simulink model "ADRC_P3DX_Madyan"  (R2024b)
settings: Solver=FixedStepAuto  StartTime=0.0  StopTime=30  FixedStep=0.01  RelTol=1e-2
libraries: simulink x1
settings Model: Creator=Dell  LastModifiedBy=MMadi
settings DebuggingCC: AlgebraicLoopMsg=none  SigSpecEnsureSampleTimeMsg=none
settings RTWCC: GPUComputeCapability=3.5

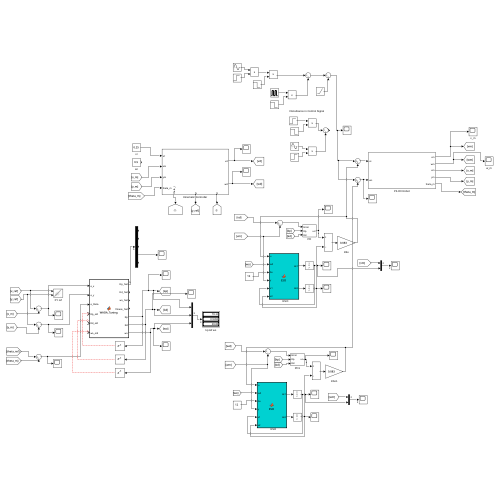
[thumbnail: Simulink's stored preview of the top-level diagram]
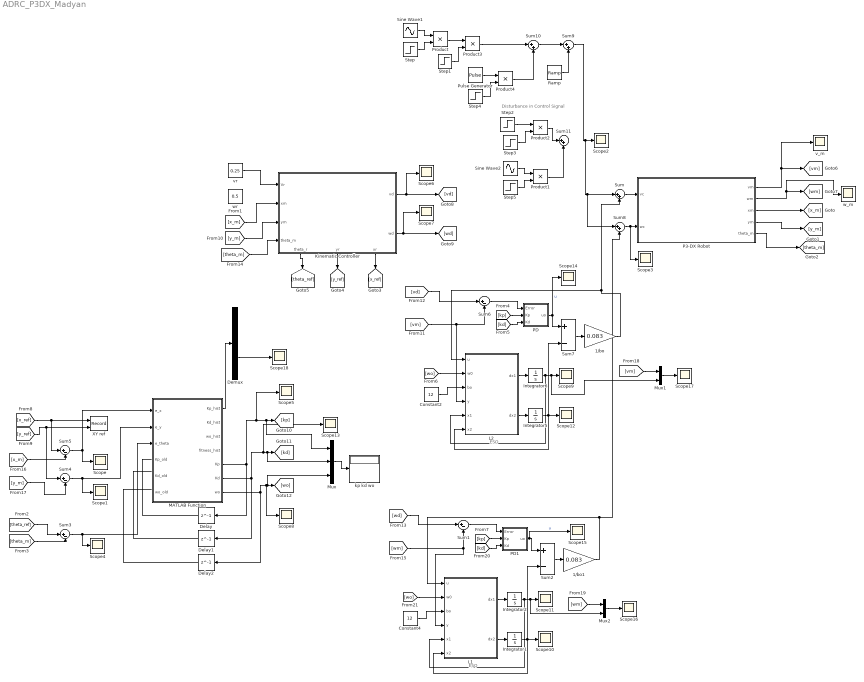
== system ADRC_P3DX_Madyan ==
  note: Disturbance in Control Signal
  note: ESO
  note: ESO
  1/bo : Gain  Gain=0.083
  1/bo1 : Gain  Gain=0.083
  Constant2 : Constant  Value=12
  Constant4 : Constant  Value=12
  Delay : Delay  DelayLength=1  InitialCondition=0
  Delay1 : Delay  DelayLength=1  InitialCondition=0
  Delay2 : Delay  DelayLength=1  InitialCondition=0
  Demux : Demux  Outputs=5
  Integrator{1..2,5..6} (4 alike) : Integrator
  Kinematic Controller : Subsystem
      settings: PortSchema="{\"entries\":[{\"content\":{\"sides\":[{\"content\":{\"connectorIds\":[\"In1\",\"In2\",\"In3\",\"In4\"]},\"type\":\"ConnectorPlacement.EquallySpacedRectSide\",\"uuid\":\"1dde3c4d-b362-4c98-bff5-173134d67a18\"},{\"content\":{\"connectorIds\":[\"Out1\",\"Out2\"],\"side\":\"RIGHT\"},\"type\":\"ConnectorPlacement.EquallySpacedRectSide\",\"uuid\":\"28a7b07a-1542-4ec6-930a-70e18e33702f\"},{\"content\":{\"side\":\"TOP\"},\"type\":\"ConnectorPlacement.EquallySpacedRectSide\",\"uuid\":\"fddfb50e-6b1f-4e7e-bd72-f809cd3d8285\"},{\"content\":{\"connectorIds\":[\"Out3\",\"Out4\",\"Out5\"],\"side\":\"BOTTOM\"},\"type\":\"ConnectorPlacement.EquallySpacedRectSide\",\"uuid\":\"0cbc9f95-9386-4a92-999a-6cc6855b0431\"}]},\"type\":\"ConnectorPlacement.EquallySpacedConnector\",\"uuid\":\"21383b85-61ab-4832-be46-2fedf08e757e\"}],\"packageUris\":[\"http://schema.mathworks.com/mf0/Connector/R2020b\"],\"version\":\"1.0\"}"
  L1 : MATLAB Function  TreatAsAtomicUnit=on
  L2 : MATLAB Function  TreatAsAtomicUnit=on
  MATLAB Function : MATLAB Function  TreatAsAtomicUnit=on
  Mux : Mux  Inputs=3
  Mux1 : Mux  Inputs=2
  Mux2 : Mux  Inputs=2
  P3-DX Robot : Subsystem
  PD : Subsystem
  PD1 : Subsystem
  Product{,1..4} (5 alike) : Product
  Pulse Generator : DiscretePulseGenerator  PulseType=Time based  Amplitude=4  Period=1  PulseWidth=35  PhaseDelay=9.7
  Ramp : simulink/Sources/Ramp  slope=1  start=25  InitialOutput=0
  Scope{,1..18} (19 alike) : Scope
  Sine Wave1 : Sin  Amplitude=4  Frequency=2  SampleTime=0
  Sine Wave2 : Sin  Amplitude=3  Frequency=2  SampleTime=0
  Step : Step  Time=3.2  SampleTime=0
  Step1 : Step  Time=15  Before=1  After=0  SampleTime=0
  Step2 : Step  Time=8  After=1.8  SampleTime=0
  Step3 : Step  Time=10  Before=1.8  After=0  SampleTime=0
  Step4 : Step  Time=23  Before=1  After=0  SampleTime=0
  Step5 : Step  Time=20  SampleTime=0
  Sum{,8..11} (5 alike) : Sum  Inputs=|++
  Sum{1,3..6} (5 alike) : Sum  Inputs=|+-
  Sum2 : Sum  Inputs=+-
  Sum7 : Sum  Inputs=+-
  XY ref : Record  FileSettingsInternal="{\"entries\":[{\"content\":{\"excelSettings\":{\"content\":{},\"type\":\"Streamout.ExcelSettings\"}},\"type\":\"Streamout.FileSettingStorage\",\"uuid\":\"\"}],\"packageUris\":[\"http:\\/\\/schema.mathworks.com\\/mf0\\/streamout_blocks\\/R2020a\"],\"version\":\"1.0\"}"  Layout=[1 1]  SignalsInternal="{\"entries\":[{\"content\":{\"signals\":[{\"content\":{\"blockPath\":[],\"dimensions\":[1],\"domain\":\"\",\"lineColor\":\"#edb120\",\"lineWidth\":2,\"port\":1,\"signalID\":1,\"signalName\":\"From8\"},\"type\":\"RecordBlkView.Signal\",\"uuid\":\"\"},{\"content\":{\"blockPath\":[],\"dimensions\":[1],\"domain\":\"\",\"lineColor\":\"#7e2f8e\",\"lineWidth\":2,\"port\":2,\"signalID\":2,\"signalName\":\"From9\"},\"type\":\"RecordBlkView.Signal\",\"uuid\":\"\"}]},\"type\":\"RecordBlkView.InputSignals\",\"uuid\":\"\"}],\"packageUris\":[\"http:\\/\\/schema.mathworks.com\\/mf0\\/streamout_blocks\\/R2020a\"],\"version\":\"1.0\"}"  VisualizationBindings="{\"xyplotplugin\":{\"info\":[{\"series\":[],\"subplotID\":1}]}}"  CompatibilityTag=XY
  kp kd wo : Display
  v_m : Scope
  vr : Constant  Value=0.25
  w_m : Scope
  wr : Constant  Value=0.5
  wires:
  [y_ref] -> Sum4/1, XY ref/2
  [x_ref] -> Sum5/1, XY ref/1
  [y_m] -> Kinematic Controller/3(ym)
  vr/1 -> Kinematic Controller/1(Vr)
  [x_m] -> Kinematic Controller/2(xm)
  [theta_m] -> Kinematic Controller/4(theta_m)
  P3-DX Robot/3(xm) -> [x_m]
  P3-DX Robot/4(ym) -> [y_m]
  P3-DX Robot/5(theta_m) -> [theta_m]
  Kinematic Controller/5(xr) -> [x_ref]
  Kinematic Controller/4(yr) -> [y_ref]
  Kinematic Controller/3(theta_r) -> [theta_ref]
  Kinematic Controller/2(wd) -> [wd], Scope7/1
  Kinematic Controller/1(vd) -> [vd], Scope6/1
  1/bo/1 -> Sum/2, L2/1(u)
  [vd] -> Sum6/1
  Integrator6/1 -> L2/5(x1), Mux1/2, Scope9/1
  Sum7/1 -> 1/bo/1
  PD/1(uo) -> Sum7/1, Scope14/1  "u"
  [vm] -> Sum6/2, L2/4(y)
  Sum6/1 -> PD/1(Error)
  Integrator5/1 -> Sum7/2, Scope12/1, L2/6(x2)
  L2/2(dx2) -> Integrator5/1
  L2/1(dx1) -> Integrator6/1
  L1/2(dx2) -> Integrator1/1
  Integrator1/1 -> Sum2/2, Scope10/1, L1/6(x2)
  [wm] -> L1/4(y), Sum1/2
  Sum1/1 -> PD1/1(Error)
  Sum2/1 -> 1/bo1/1
  Integrator2/1 -> L1/5(x1), Mux2/2, Scope11/1
  L1/1(dx1) -> Integrator2/1
  [wd] -> Sum1/1
  Constant4/1 -> L1/3(bo)
  PD1/1(uo) -> Scope15/1, Sum2/1  "u"
  1/bo1/1 -> Sum8/2, L1/1(u)
  Sum/1 -> P3-DX Robot/1(vc)
  Sum8/1 -> Scope3/1, P3-DX Robot/2(wc)
  [vm] -> Mux1/1
  Mux1/1 -> Scope17/1
  [wm] -> Mux2/1
  Mux2/1 -> Scope16/1
  Constant2/1 -> L2/3(bo)
  Sine Wave2/1 -> Product1/1
  Step5/1 -> Product1/2
  Step3/1 -> Product2/2
  Step2/1 -> Product2/1
  P3-DX Robot/1(vm) -> v_m/1, [vm]
  P3-DX Robot/2(wm) -> w_m/1, [wm]
  MATLAB Function/6(Kd) -> Scope13/1, Mux/2, [kd], Delay1/1
  MATLAB Function/7(wo) -> Scope8/1, Mux/3, [wo], Delay2/1
  MATLAB Function/5(Kp) -> Scope5/1, Mux/1, [kp], Delay/1
  [theta_ref] -> Sum3/1
  [theta_m] -> Sum3/2
  [y_m] -> Sum4/2
  [x_m] -> Sum5/2
  Sum5/1 -> Scope/1, MATLAB Function/1(e_x)
  Sum4/1 -> Scope1/1, MATLAB Function/2(e_y)
  Sum3/1 -> Scope4/1, MATLAB Function/3(e_theta)
  [kp] -> PD/2(Kp)
  [kd] -> PD/3(Kd)
  [wo] -> L2/2(w0)
  Delay/1 -> ?
  Delay1/1 -> ?
  Delay2/1 -> ?
  Mux/1 -> kp kd wo/1
  [kp] -> PD1/2(Kp)
  [kd] -> PD1/3(Kd)
  [wo] -> L1/2(w0)
  Product1/1 -> Sum11/2
  Product2/1 -> Sum11/1
  Product3/1 -> Sum10/1
  Pulse Generator/1 -> Product4/1
  Step/1 -> Product/2
  Ramp/1 -> Sum9/2
  Sum10/1 -> Sum9/1
  Product/1 -> Product3/1
  Step1/1 -> Product3/2
  Sine Wave1/1 -> Product/1
  Product4/1 -> Sum10/2
  Step4/1 -> Product4/2
  Sum9/1 -> Sum8/1, Sum/1, Scope2/1
  Demux/4 -> Scope18/1
  MATLAB Function/1(Kp_hist) -> Demux/1

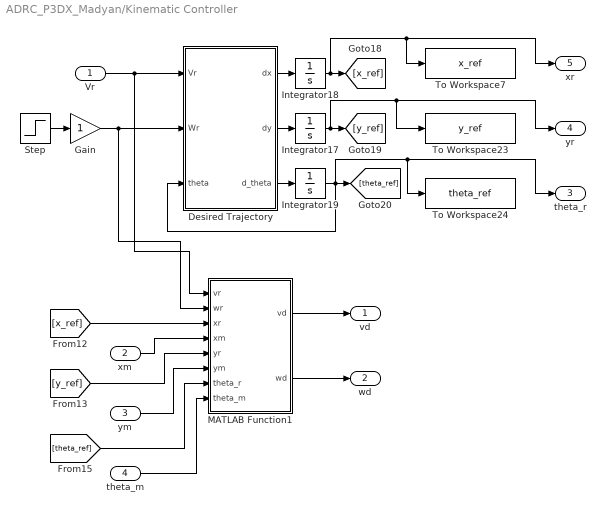
== system ADRC_P3DX_Madyan/Kinematic Controller ==
  Vr : Inport
  xm : Inport  Port=2
  ym : Inport  Port=3
  theta_m : Inport  Port=4
  " Desired Trajectory" : MATLAB Function  TreatAsAtomicUnit=on
  Gain : Gain
  Integrator17 : Integrator  InitialCondition=-0.5
  Integrator18 : Integrator
  Integrator19 : Integrator
  MATLAB Function1 : MATLAB Function  TreatAsAtomicUnit=on
  Step : Step  Time=16  Before=0.5  After=0.4  SampleTime=0
  To Workspace23 : ToWorkspace  VariableName=y_ref  SaveFormat=Timeseries  SampleTime=-1
  To Workspace24 : ToWorkspace  VariableName=theta_ref  SaveFormat=Timeseries  SampleTime=-1
  To Workspace7 : ToWorkspace  VariableName=x_ref  SaveFormat=Timeseries  SampleTime=-1
  vd : Outport
  wd : Outport  Port=2
  theta_r : Outport  Port=3
  yr : Outport  Port=4
  xr : Outport  Port=5
  wires:
  " Desired Trajectory"/3(d_theta) -> Integrator19/1
  Integrator19/1 -> theta_r/1, To Workspace24/1, " Desired Trajectory"/3(theta), [theta_ref]
  Integrator18/1 -> xr/1, To Workspace7/1, [x_ref]
  Vr/1 -> MATLAB Function1/1(vr), " Desired Trajectory"/1(Vr)
  " Desired Trajectory"/1(dx) -> Integrator18/1
  Gain/1 -> MATLAB Function1/2(wr), " Desired Trajectory"/2(Wr)
  MATLAB Function1/1(vd) -> vd/1
  MATLAB Function1/2(wd) -> wd/1
  " Desired Trajectory"/2(dy) -> Integrator17/1
  Integrator17/1 -> yr/1, To Workspace23/1, [y_ref]
  [x_ref] -> MATLAB Function1/3(xr)
  xm/1 -> MATLAB Function1/4(xm)
  [y_ref] -> MATLAB Function1/5(yr)
  ym/1 -> MATLAB Function1/6(ym)
  [theta_ref] -> MATLAB Function1/7(theta_r)
  theta_m/1 -> MATLAB Function1/8(theta_m)
  Step/1 -> Gain/1

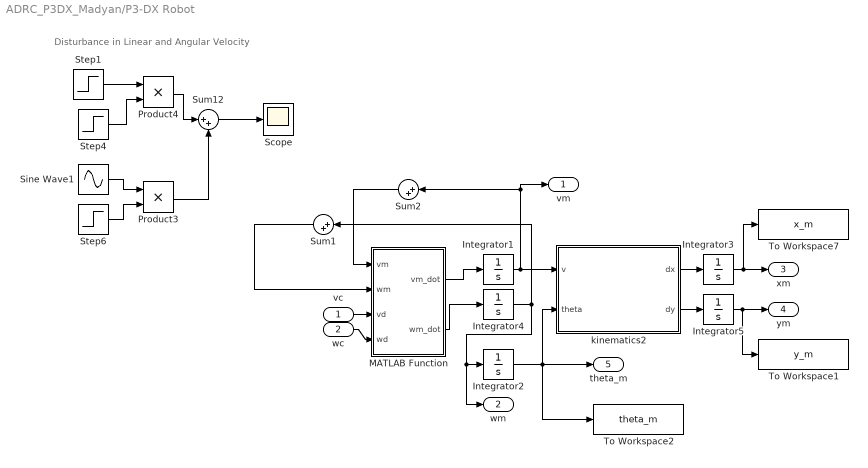
== system ADRC_P3DX_Madyan/P3-DX Robot ==
  note: Disturbance in Linear and Angular Velocity
  vc : Inport
  wc : Inport  Port=2
  Integrator{1..5} (5 alike) : Integrator
  MATLAB Function : MATLAB Function  TreatAsAtomicUnit=on
  Product3 : Product
  Product4 : Product
  Scope : Scope
  Sine Wave1 : Sin  Amplitude=4  Frequency=2  SampleTime=0
  Step1 : Step  Time=8  After=2.2  SampleTime=0
  Step4 : Step  Time=10  Before=2.2  After=0  SampleTime=0
  Step6 : Step  Time=20  SampleTime=0
  Sum1 : Sum  Inputs=|++
  Sum12 : Sum  Inputs=|++
  Sum2 : Sum  Inputs=|++
  To Workspace1 : ToWorkspace  VariableName=y_m  SaveFormat=Timeseries  SampleTime=-1
  To Workspace2 : ToWorkspace  VariableName=theta_m  SaveFormat=Timeseries  SampleTime=-1
  To Workspace7 : ToWorkspace  VariableName=x_m  SaveFormat=Timeseries  SampleTime=-1
  kinematics2 : MATLAB Function  TreatAsAtomicUnit=on
  vm : Outport
  wm : Outport  Port=2
  xm : Outport  Port=3
  ym : Outport  Port=4
  theta_m : Outport  Port=5
  wires:
  Integrator2/1 -> To Workspace2/1, theta_m/1, kinematics2/2(theta)
  MATLAB Function/1(vm_dot) -> Integrator1/1
  MATLAB Function/2(wm_dot) -> Integrator4/1
  Integrator1/1 -> kinematics2/1(v), Sum2/1, vm/1
  Integrator3/1 -> To Workspace7/1, xm/1
  Integrator4/1 -> Integrator2/1, wm/1, Sum1/1
  kinematics2/2(dy) -> Integrator5/1
  vc/1 -> MATLAB Function/3(vd)
  kinematics2/1(dx) -> Integrator3/1
  wc/1 -> MATLAB Function/4(wd)
  Integrator5/1 -> To Workspace1/1, ym/1
  Product4/1 -> Sum12/1
  Step4/1 -> Product4/2
  Step1/1 -> Product4/1
  Product3/1 -> Sum12/2
  Sine Wave1/1 -> Product3/1
  Step6/1 -> Product3/2
  Sum1/1 -> MATLAB Function/2(wm)
  Sum2/1 -> MATLAB Function/1(vm)
  Sum12/1 -> Scope/1

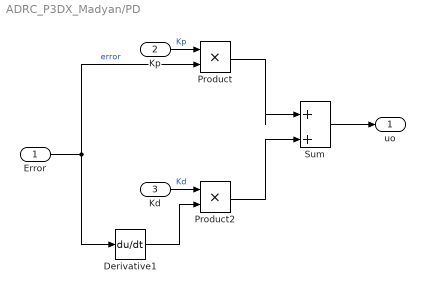
== system ADRC_P3DX_Madyan/PD ==
  Error : Inport
  Kp : Inport  Port=2
  Kd : Inport  Port=3
  Derivative1 : Derivative
  Product : Product
  Product2 : Product
  Sum : Sum  Inputs=|++
  uo : Outport
  wires:
  Derivative1/1 -> Product2/2
  Sum/1 -> uo/1
  Product/1 -> Sum/1
  Error/1 -> Derivative1/1, Product/2  "error"
  Kd/1 -> Product2/1  "Kd"
  Kp/1 -> Product/1  "Kp"
  Product2/1 -> Sum/2

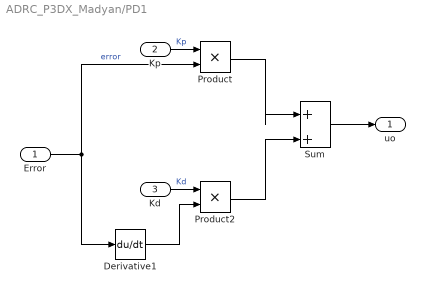
== system ADRC_P3DX_Madyan/PD1 ==
  Error : Inport
  Kp : Inport  Port=2
  Kd : Inport  Port=3
  Derivative1 : Derivative
  Product : Product
  Product2 : Product
  Sum : Sum  Inputs=|++
  uo : Outport
  wires:
  Derivative1/1 -> Product2/2
  Sum/1 -> uo/1
  Product/1 -> Sum/1
  Error/1 -> Derivative1/1, Product/2  "error"
  Kd/1 -> Product2/1  "Kd"
  Kp/1 -> Product/1  "Kp"
  Product2/1 -> Sum/2

== matlab function ADRC_P3DX_Madyan/L2 ==
  data: dx1 output; dx2 output; u input; w0 input; bo input; y input; x1 input; x2 input
function [dx1, dx2] = ESO(u, w0,bo, y, x1, x2)

%bo=[15.5311 -3.5587;
    %-3.5587 15.5311];
% l1, l2, l3 ARE THE OBSERVER GAINS IN ESO calcualated using w0
L1=2*w0;   
L2=w0^2;

e = x1-y;

dx1 = x2 + (bo * u) - (L1 * e);
dx2 = - (L2 * e);

== matlab function ADRC_P3DX_Madyan/Kinematic Controller/ Desired Trajectory ==
  data: Vr input; Wr input; theta input; dx output; dy output; d_theta output
function [dx, dy, d_theta] = desiredtraj(Vr, Wr, theta)
    dx = cos(theta) * Vr ;
    dy = sin(theta) * Vr ;
    d_theta = Wr;
    

end

== matlab function ADRC_P3DX_Madyan/Kinematic Controller/MATLAB Function1 ==
  data: vr input; wr input; xr input; vd output; xm input; yr input; ym input; theta_r input; theta_m input; wd output
function [vd, wd] = fcn(vr, wr, xr, xm, yr, ym, theta_r, theta_m)
ex = ((xr - xm) * cos(theta_m)) + ((yr - ym) * sin(theta_m));
ey = - ((xr - xm) * sin(theta_m)) + ((yr - ym) * cos(theta_m));

etheta = theta_r - theta_m;

kx = 0.8;
ky = 0.8;
kth = 0.8;

vd = (kx * ex) + (vr * cos(etheta));
wd = (ky * vr * ey ) + wr + (kth * sin(etheta));

== matlab function ADRC_P3DX_Madyan/P3-DX Robot/MATLAB Function ==
  data: vm input; vm_dot output; wm input; wm_dot output; vd input; wd input
function[vm_dot, wm_dot] = fcn(vm,wm,vd,wd)
k1 = 0.24089;
k2 = 0.2424;
k3 = -0.00093603;
k4 = 0.99629;
k5 = -0.0057256;
k6 = 1;


vm_dot = ((k3/k1) * (wm*wm)) - ((k4/k1) * vm) + (vd/k1);
wm_dot = - ((k5/k2) * (vm*wm)) - ((k6/k2) * wm) + (wd/k2);

== matlab function ADRC_P3DX_Madyan/P3-DX Robot/kinematics2 ==
  data: v input; dx output; dy output; theta input
function [dx, dy] = kinematics(v, theta)


dx =  v .* cos(theta);
dy =  v .* sin(theta);

== matlab function ADRC_P3DX_Madyan/L1 ==
  data: dx1 output; dx2 output; u input; w0 input; bo input; y input; x1 input; x2 input
function [dx1,dx2] =ESO(u,w0,bo, y, x1,x2)
%bo=[15.5311 -3.5587;
    %-3.5587 15.5311];
% l1, l2, l3 ARE THE OBSERVER GAINS IN ESO calcualated using w0
L1=2*w0;   
L2=w0^2;

e = x1-y;

dx1 = x2 + (bo * u) - (L1 * e);
dx2 = - (L2 * e);

== matlab function ADRC_P3DX_Madyan/MATLAB Function ==
  settings: updateMethod=DISCRETE
  data: Kp_hist output; Kd_hist output; wo_hist output; fitness_hist output; e_x input; Kp output; e_y input; e_theta input; Kd output; wo output; Kp_old input; Kd_old input; wo_old input


%{
function [Kp_hist, Kd_hist, wo_hist, fitness_hist, Kp, Kd, wo] = GA_Tuning(e_x, e_y, e_theta, Kp_old, Kd_old, wo_old)

    % Number of GA iterations per update
    num_generations = 5;
    pop_size = 10;

    % Parameter search space
    lb = [0, 0, 0];
    ub = [100, 1, 50];

    % Objective function
    fitnessFunction = @(params) sum(e_x.^2 + e_y.^2 + e_theta.^2);

    % Initialize population randomly
    population = lb + (ub - lb) .* rand(pop_size, 3);

    % History arrays
    Kp_hist = zeros(num_generations, 1);
    Kd_hist = zeros(num_generations, 1);
    wo_hist = zeros(num_generations, 1);
    fitness_hist = zeros(num_generations, 1);

    for gen = 1:num_generations
        % Evaluate fitness
        fitness_vec = arrayfun(@(i) fitnessFunction(population(i, :)), 1:pop_size);
        
        % Best individual this generation
        [fitness, bestIdx] = min(fitness_vec);
        bestParams = population(bestIdx, :);

        % Save history
        Kp_hist(gen) = bestParams(1);
        Kd_hist(gen) = bestParams(2);
        wo_hist(gen) = bestParams(3);
        fitness_hist(gen) = fitness;

        % Crossover and mutation
        for i = 1:pop_size
            if rand < 0.7  % Crossover rate
                parentIdx = randi([1, pop_size]);
                population(i, :) = (population(i, :) + population(parentIdx, :)) / 2;
            end
            if rand < 0.2  % Mutation rate
                mutation = (ub - lb) .* (rand(1, 3) - 0.5) * 0.1;
                population(i, :) = population(i, :) + mutation;
            end
        end

        % Keep within bounds
        population = max(min(population, ub), lb);
    end

    % Output best found in final generation
    Kp = bestParams(1);
    Kd = bestParams(2);
    wo = bestParams(3);

end
%}

%{
function [Kp_hist, Kd_hist, wo_hist, fitness_hist, Kp, Kd, wo] = GA_Tuning(e_x, e_y, e_theta, Kp_old, Kd_old, wo_old)

    % Number of GA iterations per update
    num_generations = 5;
    pop_size = 10;

    % Parameter search space
    lb = [0, 0, 0];
    ub = [100, 1, 50];

    % Objective function (fitness)
    fitnessFunction = @(params) sum(e_x.^2 + e_y.^2 + e_theta.^2);

    % Initialize population randomly
    population = lb + (ub - lb) .* rand(pop_size, 3);

    % Constants for adaptation
    k1 = 1.0;  % For crossover adaptation
    k2 = 0.9;  % Default crossover if not adapted
    k3 = 1.0;  % For mutation adaptation
    k4 = 0.1;  % Default mutation if not adapted

    % History arrays
    Kp_hist = zeros(num_generations, 1);
    Kd_hist = zeros(num_generations, 1);
    wo_hist = zeros(num_generations, 1);
    fitness_hist = zeros(num_generations, 1);

    for gen = 1:num_generations
        % Evaluate fitness
        fitness_vec = arrayfun(@(i) fitnessFunction(population(i, :)), 1:pop_size);

        % Best individual this generation
        [fitness, bestIdx] = min(fitness_vec);
        bestParams = population(bestIdx, :);

        % Save history
        Kp_hist(gen) = bestParams(1);
        Kd_hist(gen) = bestParams(2);
        wo_hist(gen) = bestParams(3);
        fitness_hist(gen) = fitness;

        favg = mean(fitness_vec);
        fmax = max(fitness_vec);

        % Crossover and mutation (adaptive version)
        new_population = zeros(size(population));
        for i = 1:pop_size
            % Select parents
            parent1 = population(i, :);
            idx2 = randi([1, pop_size]);
            parent2 = population(idx2, :);

            % Crossover probability (adaptive)
            f = max(fitness_vec(i), fitness_vec(idx2));
            if f >= favg
                Pc = k1 * (fmax - f) / (fmax - favg);
            else
                Pc = k2;
            end
            Pc = min(max(Pc, 0), 1);

            child = parent1;
            if rand < Pc
                % Single point crossover
                cp = randi([1, 2]); % Crossover point (between 1 and 2)
                child(1:cp) = parent2(1:cp);
            end

            % Mutation probability (adaptive)
            f_child = fitnessFunction(child);
            if f_child >= favg
                Pm = k3 * (fmax - f_child) / (fmax - favg);
            else
                Pm = k4;
            end
            Pm = min(max(Pm, 0), 1);

            % Mutation operation
            if rand < Pm
                mutationPoint = randi([1, 3]);
                mutationAmount = (ub(mutationPoint) - lb(mutationPoint)) * (rand - 0.5) * 0.2;
                child(mutationPoint) = child(mutationPoint) + mutationAmount;
            end

            % Store child
            new_population(i, :) = child;
        end

        % Keep within bounds
        population = max(min(new_population, ub), lb);
    end

    % Output best found in final generation
    Kp = bestParams(1);
    Kd = bestParams(2);
    wo = bestParams(3);

end
%}


function [Kp_hist, Kd_hist, wo_hist, fitness_hist, Kp, Kd, wo] = MPAGA_Tuning(e_x, e_y, e_theta, Kp_old, Kd_old, wo_old)

    % Settings
    num_generations = 10;
    pop_size = 10;
    num_pops = 3;   % Number of sub-populations

    % Search space
    lb = [0, 0, 0];
    ub = [100, 1, 50];

    % Objective function
    fitnessFunction = @(params) sum(e_x.^2 + e_y.^2 + e_theta.^2);

    % Preallocate populations and fitness arrays
    populations = zeros(pop_size, 3, num_pops);
    fitnesses = zeros(pop_size, num_pops);

    % Initialize populations
    for p = 1:num_pops
        populations(:,:,p) = lb + (ub - lb) .* rand(pop_size, 3);
        for i = 1:pop_size
            fitnesses(i,p) = fitnessFunction(populations(i,:,p));
        end
    end

    % Adaptive constants
    k1 = 1.0; k2 = 0.9;
    k3 = 1.0; k4 = 0.1;

    % History arrays
    Kp_hist = zeros(num_generations, 1);
    Kd_hist = zeros(num_generations, 1);
    wo_hist = zeros(num_generations, 1);
    fitness_hist = zeros(num_generations, 1);

    % Initialize bestParams (important for code generation!)
    bestParams = zeros(1,3);
    allBestFitness = inf;

    for gen = 1:num_generations

        % Evolution within each population
        for p = 1:num_pops
            pop = populations(:,:,p);
            fit = fitnesses(:,p);

            favg = mean(fit);
            fmax = max(fit);

            new_pop = zeros(size(pop));
            for i = 1:pop_size
                % Select two parents randomly
                idx1 = randi([1, pop_size]);
                idx2 = randi([1, pop_size]);
                parent1 = pop(idx1, :);
                parent2 = pop(idx2, :);

                % Adaptive crossover probability
                f = max(fit(idx1), fit(idx2));
                if f >= favg
                    Pc = k1 * (fmax - f) / (fmax - favg);
                else
                    Pc = k2;
                end
                Pc = min(max(Pc, 0), 1);

                % Crossover
                child = parent1;
                if rand < Pc
                    cp = randi([1, 2]);
                    child(1:cp) = parent2(1:cp);
                end

                % Adaptive mutation probability
                f_child = fitnessFunction(child);
                if f_child >= favg
                    Pm = k3 * (fmax - f_child) / (fmax - favg);
                else
                    Pm = k4;
                end
                Pm = min(max(Pm, 0), 1);

                % Mutation
                if rand < Pm
                    mutationPoint = randi([1, 3]);
                    mutationAmount = (ub(mutationPoint) - lb(mutationPoint)) * (rand - 0.5) * 0.2;
                    child(mutationPoint) = child(mutationPoint) + mutationAmount;
                end

                % Store child
                new_pop(i,:) = child;
            end

            % Bounds check
            new_pop = max(min(new_pop, ub), lb);

            % Update population and fitness
            populations(:,:,p) = new_pop;
            for i = 1:pop_size
                fitnesses(i,p) = fitnessFunction(new_pop(i,:));
            end
        end

        % Immigration step
        for p = 1:num_pops
            next_p = mod(p, num_pops) + 1;
            [~, bestIdx] = min(fitnesses(:,p));
            [~, worstIdx] = max(fitnesses(:,next_p));
            populations(worstIdx,:,next_p) = populations(bestIdx,:,p);
            fitnesses(worstIdx,next_p) = fitnesses(bestIdx,p);
        end

        % Find best across all populations
        for p = 1:num_pops
            [minFit, idx] = min(fitnesses(:,p));
            if minFit < allBestFitness
                allBestFitness = minFit;
                bestParams = populations(idx,:,p);
            end
        end

        % Save history
        Kp_hist(gen) = bestParams(1);
        Kd_hist(gen) = bestParams(2);
        wo_hist(gen) = bestParams(3);
        fitness_hist(gen) = allBestFitness;
    end

    % Output
    Kp = bestParams(1);
    Kd = bestParams(2);
    wo = bestParams(3);

end

%}


%{
function [Kp_hist, Kd_hist, wo_hist, fitness_hist, Kp, Kd, wo] = AGA_Tuning(e_x, e_y, e_theta, Kp_old, Kd_old, wo_old)

    % Number of GA iterations per update
    num_generations = 5;
    pop_size = 10;

    % Parameter search space
    lb = [0, 0, 0];
    ub = [100, 1, 50];

    % Objective function (fitness)
    fitnessFunction = @(params) sum(e_x.^2 + e_y.^2 + e_theta.^2);

    % Initialize population randomly
    population = lb + (ub - lb) .* rand(pop_size, 3);

    % Constants for adaptation
    k1 = 1.0;  % For crossover adaptation
    k2 = 0.9;  % Default crossover if not adapted
    k3 = 1.0;  % For mutation adaptation
    k4 = 0.1;  % Default mutation if not adapted

    % History arrays
    Kp_hist = zeros(num_generations, 1);
    Kd_hist = zeros(num_generations, 1);
    wo_hist = zeros(num_generations, 1);
    fitness_hist = zeros(num_generations, 1);

    for gen = 1:num_generations
        % Evaluate fitness
        fitness_vec = arrayfun(@(i) fitnessFunction(population(i, :)), 1:pop_size);

        % Best individual this generation
        [fitness, bestIdx] = min(fitness_vec);
        bestParams = population(bestIdx, :);

        % Save history
        Kp_hist(gen) = bestParams(1);
        Kd_hist(gen) = bestParams(2);
        wo_hist(gen) = bestParams(3);
        fitness_hist(gen) = fitness;

        favg = mean(fitness_vec);
        fmax = max(fitness_vec);

        % Crossover and mutation (adaptive version)
        new_population = zeros(size(population));
        for i = 1:pop_size
            % Select parents
            parent1 = population(i, :);
            idx2 = randi([1, pop_size]);
            parent2 = population(idx2, :);

            % Crossover probability (adaptive)
            f = max(fitness_vec(i), fitness_vec(idx2));
            if f >= favg
                Pc = k1 * (fmax - f) / (fmax - favg);
            else
                Pc = k2;
            end
            Pc = min(max(Pc, 0), 1);

            child = parent1;
            if rand < Pc
                % Single point crossover
                cp = randi([1, 2]); % Crossover point (between 1 and 2)
                child(1:cp) = parent2(1:cp);
            end

            % Mutation probability (adaptive)
            f_child = fitnessFunction(child);
            if f_child >= favg
                Pm = k3 * (fmax - f_child) / (fmax - favg);
            else
                Pm = k4;
            end
            Pm = min(max(Pm, 0), 1);

            % Mutation operation
            if rand < Pm
                mutationPoint = randi([1, 3]);
                mutationAmount = (ub(mutationPoint) - lb(mutationPoint)) * (rand - 0.5) * 0.2;
                child(mutationPoint) = child(mutationPoint) + mutationAmount;
            end

            % Store child
            new_population(i, :) = child;
        end

        % Keep within bounds
        population = max(min(new_population, ub), lb);
    end

    % Output best found in final generation
    Kp = bestParams(1);
    Kd = bestParams(2);
    wo = bestParams(3);

end
%}


%{
function [Kp_hist, Kd_hist, wo_hist, fitness_hist, Kp, Kd, wo] = DE_Tuning(e_x, e_y, e_theta, Kp_old, Kd_old, wo_old)

    num_generations = 5;
    pop_size = 10;
    F = 0.8;        % Mutation factor
    CR = 0.9;       % Crossover rate
    lb = [0, 0, 0];
    ub = [100, 1, 50];

    fitnessFunction = @(params) sum(e_x.^2 + e_y.^2 + e_theta.^2);

    population = lb + (ub - lb) .* rand(pop_size, 3);
    fitness_vec = arrayfun(@(i) fitnessFunction(population(i, :)), 1:pop_size);

    Kp_hist = zeros(num_generations, 1);
    Kd_hist = zeros(num_generations, 1);
    wo_hist = zeros(num_generations, 1);
    fitness_hist = zeros(num_generations, 1);

    for gen = 1:num_generations
        for i = 1:pop_size
            % Mutation
            idxs = randperm(pop_size, 3);
            while any(idxs == i)
                idxs = randperm(pop_size, 3);
            end
            a = population(idxs(1), :);
            b = population(idxs(2), :);
            c = population(idxs(3), :);
            mutant = a + F * (b - c);

            % Crossover
            trial = population(i, :);
            for j = 1:3
                if rand < CR
                    trial(j) = mutant(j);
                end
            end

            % Bounds check
            trial = max(min(trial, ub), lb);

            % Selection
            trial_fitness = fitnessFunction(trial);
            if trial_fitness < fitness_vec(i)
                population(i, :) = trial;
                fitness_vec(i) = trial_fitness;
            end
        end

        [fitness, bestIdx] = min(fitness_vec);
        bestParams = population(bestIdx, :);
        Kp_hist(gen) = bestParams(1);
        Kd_hist(gen) = bestParams(2);
        wo_hist(gen) = bestParams(3);
        fitness_hist(gen) = fitness;
    end

    Kp = bestParams(1);
    Kd = bestParams(2);
    wo = bestParams(3);
end
%}


%{
function [Kp_hist, Kd_hist, wo_hist, fitness_hist, Kp, Kd, wo] = CS_Tuning(e_x, e_y, e_theta, Kp_old, Kd_old, wo_old)

    num_generations = 5;
    n = 10;  % number of nests
    pa = 0.25;  % discovery rate of alien eggs
    lb = [0, 0, 0];
    ub = [100, 1, 50];

    fitnessFunction = @(params) sum(e_x.^2 + e_y.^2 + e_theta.^2);

    nests = lb + (ub - lb) .* rand(n, 3);
    fitness = arrayfun(@(i) fitnessFunction(nests(i, :)), 1:n);

    Kp_hist = zeros(num_generations, 1);
    Kd_hist = zeros(num_generations, 1);
    wo_hist = zeros(num_generations, 1);
    fitness_hist = zeros(num_generations, 1);

    for gen = 1:num_generations
        for i = 1:n
            % Lévy flight
            step_size = 0.01 * randn(1, 3);
            new_nest = nests(i, :) + step_size .* randn(1, 3);
            new_nest = max(min(new_nest, ub), lb);

            new_fitness = fitnessFunction(new_nest);
            if new_fitness < fitness(i)
                nests(i, :) = new_nest;
                fitness(i) = new_fitness;
            end
        end

        % Abandon some nests
        abandon = rand(n, 1) < pa;
        for i = 1:n
            if abandon(i)
                nests(i, :) = lb + (ub - lb) .* rand(1, 3);
                fitness(i) = fitnessFunction(nests(i, :));
            end
        end

        [fit_best, idx] = min(fitness);
        bestParams = nests(idx, :);
        Kp_hist(gen) = bestParams(1);
        Kd_hist(gen) = bestParams(2);
        wo_hist(gen) = bestParams(3);
        fitness_hist(gen) = fit_best;
    end

    Kp = bestParams(1);
    Kd = bestParams(2);
    wo = bestParams(3);
end
%}


%{
function [Kp_hist, Kd_hist, wo_hist, fitness_hist, Kp, Kd, wo] = PSO_Tuning(e_x, e_y, e_theta, ~, ~, ~)
    num_generations = 5;
    pop_size = 10;
    dim = 3;
    lb = [0, 0, 0];
    ub = [100, 1, 50];
    
    fitnessFunction = @(params) sum(e_x.^2 + e_y.^2 + e_theta.^2);

    % Initialize
    pos = lb + (ub - lb) .* rand(pop_size, dim);
    vel = zeros(pop_size, dim);
    pbest = pos;
    pbest_val = arrayfun(@(i) fitnessFunction(pos(i,:)), 1:pop_size);
    [gbest_val, idx] = min(pbest_val);
    gbest = pbest(idx, :);

    Kp_hist = zeros(num_generations, 1);
    Kd_hist = zeros(num_generations, 1);
    wo_hist = zeros(num_generations, 1);
    fitness_hist = zeros(num_generations, 1);

    for gen = 1:num_generations
        for i = 1:pop_size
            r1 = rand(1, dim);
            r2 = rand(1, dim);
            vel(i,:) = 0.5*vel(i,:) + 1.5*r1.*(pbest(i,:)-pos(i,:)) + 1.5*r2.*(gbest-pos(i,:));
            pos(i,:) = pos(i,:) + vel(i,:);
            pos(i,:) = max(min(pos(i,:), ub), lb);
            
            fit = fitnessFunction(pos(i,:));
            if fit < pbest_val(i)
                pbest(i,:) = pos(i,:);
                pbest_val(i) = fit;
            end
        end
        
        [gbest_val, idx] = min(pbest_val);
        gbest = pbest(idx, :);

        % Log best
        Kp_hist(gen) = gbest(1);
        Kd_hist(gen) = gbest(2);
        wo_hist(gen) = gbest(3);
        fitness_hist(gen) = gbest_val;
    end

    Kp = gbest(1);
    Kd = gbest(2);
    wo = gbest(3);
end
%}


%{
function [Kp_hist, Kd_hist, wo_hist, fitness_hist, Kp, Kd, wo] = GWO_Tuning(e_x, e_y, e_theta)
    num_generations = 5;
    pop_size = 10;
    dim = 3;
    lb = [0, 0, 0];
    ub = [100, 1, 50];
    fitnessFunction = @(params) sum(e_x.^2 + e_y.^2 + e_theta.^2);

    % Initialize positions
    Positions = lb + (ub - lb) .* rand(pop_size, dim);
    Alpha_pos = zeros(1, dim);
    Alpha_score = inf;
    Beta_pos = zeros(1, dim);
    Beta_score = inf;
    Delta_pos = zeros(1, dim);
    Delta_score = inf;

    Kp_hist = zeros(num_generations, 1);
    Kd_hist = zeros(num_generations, 1);
    wo_hist = zeros(num_generations, 1);
    fitness_hist = zeros(num_generations, 1);

    for gen = 1:num_generations
        for i = 1:pop_size
            % Boundary check
            Positions(i,:) = max(min(Positions(i,:), ub), lb);
            fitness = fitnessFunction(Positions(i,:));

            if fitness < Alpha_score
                Alpha_score = fitness;
                Alpha_pos = Positions(i,:);
            elseif fitness < Beta_score
                Beta_score = fitness;
                Beta_pos = Positions(i,:);
            elseif fitness < Delta_score
                Delta_score = fitness;
                Delta_pos = Positions(i,:);
            end
        end

        a = 2 - gen * (2 / num_generations); % a decreases linearly from 2 to 0

        for i = 1:pop_size
            for j = 1:dim
                r1 = rand();
                r2 = rand();

                A1 = 2 * a * r1 - a;
                C1 = 2 * r2;

                D_alpha = abs(C1 * Alpha_pos(j) - Positions(i,j));
                X1 = Alpha_pos(j) - A1 * D_alpha;

                r1 = rand();
                r2 = rand();

                A2 = 2 * a * r1 - a;
                C2 = 2 * r2;

                D_beta = abs(C2 * Beta_pos(j) - Positions(i,j));
                X2 = Beta_pos(j) - A2 * D_beta;

                r1 = rand();
                r2 = rand();

                A3 = 2 * a * r1 - a;
                C3 = 2 * r2;

                D_delta = abs(C3 * Delta_pos(j) - Positions(i,j));
                X3 = Delta_pos(j) - A3 * D_delta;

                Positions(i,j) = (X1 + X2 + X3) / 3;
            end
        end

        % Log best
        Kp_hist(gen) = Alpha_pos(1);
        Kd_hist(gen) = Alpha_pos(2);
        wo_hist(gen) = Alpha_pos(3);
        fitness_hist(gen) = Alpha_score;
    end

    Kp = Alpha_pos(1);
    Kd = Alpha_pos(2);
    wo = Alpha_pos(3);
end
%}


%{
function [Kp_hist, Kd_hist, wo_hist, fitness_hist, Kp, Kd, wo] = ABC_Tuning(e_x, e_y, e_theta)
    % Parameters
    num_generations = 5;
    pop_size = 10;
    FoodNumber = pop_size / 2;
    dim = 3;
    lb = [0, 0, 0];
    ub = [100, 1, 50];
    limit = 5;

    % Objective function
    fitnessFunction = @(params) sum(e_x.^2 + e_y.^2 + e_theta.^2); % You can replace this with your own cost

    % Initialization
    Foods = lb + (ub - lb) .* rand(FoodNumber, dim);
    f = arrayfun(@(i) fitnessFunction(Foods(i,:)), 1:FoodNumber);
    trial = zeros(FoodNumber,1);

    % Histories
    Kp_hist = zeros(num_generations, 1);
    Kd_hist = zeros(num_generations, 1);
    wo_hist = zeros(num_generations, 1);
    fitness_hist = zeros(num_generations, 1);

    for gen = 1:num_generations
        %% Employed Bee Phase
        for i = 1:FoodNumber
            phi = rand(1, dim) * 2 - 1;
            k = randi([1, FoodNumber]);
            while k == i
                k = randi([1, FoodNumber]);
            end
            vi = Foods(i,:) + phi .* (Foods(i,:) - Foods(k,:));
            vi = max(min(vi, ub), lb);  % Apply bounds

            fi = fitnessFunction(vi);
            if fi < f(i)
                Foods(i,:) = vi;
                f(i) = fi;
                trial(i) = 0;
            else
                trial(i) = trial(i) + 1;
            end
        end

        %% Onlooker Bee Phase
        fitness_inv = 1 ./ (1 + f);  % Convert cost to fitness
        prob = fitness_inv / sum(fitness_inv);
        i = 1;
        t = 0;
        while t < FoodNumber
            if rand < prob(i)
                t = t + 1;
                phi = rand(1, dim) * 2 - 1;
                k = randi([1, FoodNumber]);
                while k == i
                    k = randi([1, FoodNumber]);
                end
                vi = Foods(i,:) + phi .* (Foods(i,:) - Foods(k,:));
                vi = max(min(vi, ub), lb);

                fi = fitnessFunction(vi);
                if fi < f(i)
                    Foods(i,:) = vi;
                    f(i) = fi;
                    trial(i) = 0;
                else
                    trial(i) = trial(i) + 1;
                end
            end
            i = mod(i, FoodNumber) + 1;
        end

        %% Scout Bee Phase
        for i = 1:FoodNumber
            if trial(i) > limit
                Foods(i,:) = lb + (ub - lb) .* rand(1, dim);
                f(i) = fitnessFunction(Foods(i,:));
                trial(i) = 0;
            end
        end

        %% Memorize the best solution
        [best_fit, best_idx] = min(f);
        best_sol = Foods(best_idx, :);
        Kp_hist(gen) = best_sol(1);
        Kd_hist(gen) = best_sol(2);
        wo_hist(gen) = best_sol(3);
        fitness_hist(gen) = best_fit;
    end

    % Return best solution
    Kp = Kp_hist(end);
    Kd = Kd_hist(end);
    wo = wo_hist(end);
end
%}


%{
function [Kp_hist, Kd_hist, wo_hist, fitness_hist, Kp, Kd, wo] = SFOA_Tuning(e_x, e_y, e_theta, Kp_old, Kd_old, wo_old)

    % Parameters
    num_generations = 5;
    pop_size = 10;
    dim = 3; % [Kp, Kd, wo]
    lb = [0, 0, 0];
    ub = [100, 1, 50];
    Gp = 0.5; % Probability to switch between exploration and exploitation

    % Fitness function
    fitnessFunction = @(params) sum(e_x.^2 + e_y.^2 + e_theta.^2);

    % Initialization
    population = repmat(lb, pop_size, 1) + rand(pop_size, dim) .* (repmat(ub - lb, pop_size, 1));
    fitness_vec = arrayfun(@(i) fitnessFunction(population(i,:)), 1:pop_size)';

    Kp_hist = zeros(num_generations, 1);
    Kd_hist = zeros(num_generations, 1);
    wo_hist = zeros(num_generations, 1);
    fitness_hist = zeros(num_generations, 1);

    for gen = 1:num_generations
        for i = 1:pop_size
            r = rand;
            if r < Gp  % Exploration
                p = randi(dim);
                k1 = randi(pop_size);
                k2 = randi(pop_size);
                while k1 == i, k1 = randi(pop_size); end
                while k2 == i || k2 == k1, k2 = randi(pop_size); end

                A1 = 2 * rand - 1;
                A2 = 2 * rand - 1;
                E_t = (num_generations - gen) / num_generations;
                Y = population(i, :);
                Y(p) = E_t * Y(p) + A1 * (population(k1, p) - Y(p)) + A2 * (population(k2, p) - Y(p));
            else  % Exploitation
                [~, bestIdx] = min(fitness_vec);
                best = population(bestIdx, :);
                d1 = best - population(randi(pop_size), :);
                d2 = best - population(randi(pop_size), :);
                r1 = rand;
                r2 = rand;
                Y = population(i, :) + r1 * d1 + r2 * d2;

                % Regeneration if it's the last agent
                if i == pop_size
                    Y = exp(-gen * pop_size / num_generations) * population(i, :);
                end
            end

            % Bounds check
            Y = max(min(Y, ub), lb);

            % Fitness evaluation
            Y_fitness = fitnessFunction(Y);
            if Y_fitness < fitness_vec(i)
                population(i, :) = Y;
                fitness_vec(i) = Y_fitness;
            end
        end

        [fitness, bestIdx] = min(fitness_vec);
        bestParams = population(bestIdx, :);
        Kp_hist(gen) = bestParams(1);
        Kd_hist(gen) = bestParams(2);
        wo_hist(gen) = bestParams(3);
        fitness_hist(gen) = fitness;
    end

    Kp = bestParams(1);
    Kd = bestParams(2);
    wo = bestParams(3);
end
%}


%{
function [Kp_hist, Kd_hist, wo_hist, fitness_hist, Kp, Kd, wo] = WAOA_Tuning(e_x, e_y, e_theta, Kp_old, Kd_old, wo_old)

    % Parameters
    num_generations = 5;
    pop_size = 10;
    dim = 3; % [Kp, Kd, wo]
    lb = [0, 0, 0];
    ub = [100, 1, 50];

    % Fitness function (currently independent of Kp/Kd/wo - placeholder)
    fitness = @(params) sum(e_x.^2 + e_y.^2 + e_theta.^2);

    % Initialize population matrix
    X = zeros(pop_size, dim);
    for i = 1:dim
        X(:,i) = lb(i) + rand(pop_size,1).*(ub(i)-lb(i));
    end

    % Initialize fitness values
    fit = zeros(pop_size, 1);
    for i = 1:pop_size
        L = X(i,:);
        fit(i) = fitness(L);
    end

    % Initialize best fitness and solution
    [fbest, bestIdx] = min(fit);
    Xbest = X(bestIdx, :);

    % Initialize logs
    Kp_hist = zeros(num_generations, 1);
    Kd_hist = zeros(num_generations, 1);
    wo_hist = zeros(num_generations, 1);
    fitness_hist = zeros(num_generations, 1);

    % Main loop
    for t = 1:num_generations
        SW = Xbest;  % strongest walrus (best known solution)

        for i = 1:pop_size
            %% Phase 1: Feeding Strategy (Exploration)
            I = round(1 + rand());
            X_P1 = X(i,:) + rand(1,dim) .* (SW - I * X(i,:));
            X_P1 = max(min(X_P1, ub), lb);

            F_P1 = fitness(X_P1);
            if F_P1 < fit(i)
                X(i,:) = X_P1;
                fit(i) = F_P1;
            end

            %% Phase 2: Migration
            I = round(1 + rand());
            K = randperm(pop_size);
            K(K == i) = [];
            X_K = X(K(1),:);
            F_RAND = fit(K(1));

            if fit(i) > F_RAND
                X_P2 = X(i,:) + rand() * (X_K - I * X(i,:));
            else
                X_P2 = X(i,:) + rand() * (X(i,:) - X_K);
            end

            X_P2 = max(min(X_P2, ub), lb);
            F_P2 = fitness(X_P2);
            if F_P2 < fit(i)
                X(i,:) = X_P2;
                fit(i) = F_P2;
            end

            %% Phase 3: Escaping & Fighting Against Predators (Exploitation)
            LO_LOCAL = lb ./ t;
            HI_LOCAL = ub ./ t;
            X_P3 = X(i,:) + LO_LOCAL + rand() * (HI_LOCAL - LO_LOCAL);
            X_P3 = max(min(X_P3, ub), lb);

            F_P3 = fitness(X_P3);
            if F_P3 < fit(i)
                X(i,:) = X_P3;
                fit(i) = F_P3;
            end
        end

        % Update best solution of the current generation
        [curr_best, curr_bestIdx] = min(fit);
        if curr_best < fbest
            fbest = curr_best;
            Xbest = X(curr_bestIdx, :);
        end

        % Record history
        Kp_hist(t) = Xbest(1);
        Kd_hist(t) = Xbest(2);
        wo_hist(t) = Xbest(3);
        fitness_hist(t) = fbest;
    end

    % Final best parameters
    Kp = Xbest(1);
    Kd = Xbest(2);
    wo = Xbest(3);
end
%}
